simulink model "Sat_Int_test"  (Simulink 7.3)
settings: Solver=ode45  StartTime=0.0  StopTime=10.0  RelTol=1e-3
settings Model: Creator=MD710  LastModifiedBy=MD710
settings DebuggingCC: SaveWithParameterizedLinksMsg=none  SolverPrmCheckMsg=none  MultiTaskDSMMsg=warning  MultiTaskCondExecSysMsg=none  FcnCallInpInsideContextMsg=Enable All  StrictBusMsg=None
settings HardwareCC: TargetHWDeviceType=32-bit Generic
settings RTWCC: IncludeERTFirstTime=on
settings GRTTargetCC: TargetFcnLib=ansi_tfl_tmw.mat

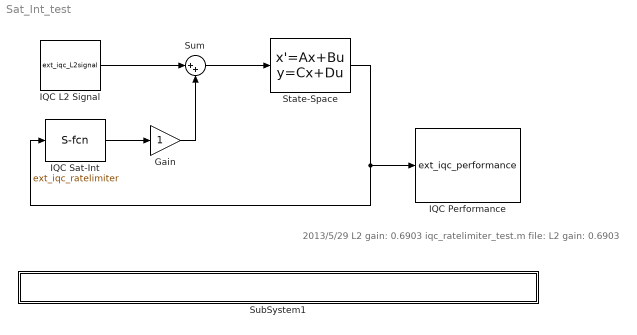
== system Sat_Int_test ==
  note: 2013/5/29 L2 gain: 0.6903
      | iqc_ratelimiter_test.m file: L2 gain: 0.6903
  Gain : Gain
  IQC L2 Signal : M-S-Function  FunctionName=ext_iqc_L2signal  Parameters=sig_size,sam_time,sig_type,tru_time,sig_amp,sig_fre,user_cus  mask(IQC L2 signal(ver:0.1)){sig_size=1, sam_time=0, sig_type=Step, tru_time=10, sig_amp=1, sig_fre=1, user_cus='2*exp(3*t)'}
      mask prompts: sig_size "Signal Dimension:(Default: 1)"; sam_time "Sample Time:(Default: 0)"; sig_type "Signal Type:"; tru_time "Truncation Time:"; sig_amp "Maximum Amplitude:"; sig_fre "Frequency:"; user_cus "Custom:"
      mask help:
      | Important:
      | In IQC procedure step (as commond iqc_gain_tbx, the task is get
      | L2 gain value), regardless of the user to choose which option (ex sine...),
      | here regarded as generalized L2 signal.
      mask StyleString: edit,edit,popup(Step|Square wave|Sine wave|Custom|Random|External),edit,edit,edit,edit
      mask CallbackString: ||iqc_block_cho(gcb,'L2signal_type')||||
      mask TabNameString: Generalized Parameters,Generalized Parameters,Simulink Parameters,Simulink Parameters,Simulink Parameters,Simulink Parameters,Simulink Parameters
      mask Display: plot(0:0.1:10,[sin(0:0.1:6.2) zeros(1,38)])
  IQC Performance : M-S-Function  FunctionName=ext_iqc_performance  Parameters=imp_met,save_lin_com,isiqcbode,fre_ran,uselmitool,lmi_par  mask(IQC Performance(ver:0.1)){imp_met=Only Calculation, save_lin_com=off, isiqcbode=off, fre_ran='', uselmitool=lmilab, lmi_par=''}
      mask prompts: imp_met "Implementation Methods"; save_lin_com "Save the Linear File and Command File"; isiqcbode "Display IQC Bode Figure"; fre_ran "Frequency Range:(Default: empty)"; uselmitool "LMI Tool:"; lmi_par "Parameter:(if empty use define)"
      mask help:
      | Important:
      | In IQC toolbox calculate step (as commond iqc_gain_tbx, the task is get
      | L2 gain value), regardless of the user to connect any signal input(Even if
      | not a signal), here regarded as generalized L2 signal.
      |
      | Example 1: setlmioptions('',[0 200 0 0 777])
      | the block parameter is
      | LMI Tool: lmilab
      | Parameter:
      |        [0 200 0 0 777]
      |
      | Example 2: setlmioptions('yalmip','solver','sdpt3','verbose',1)
      | the block parameter is
      | LMI Tool: yalmip
      | Parameter:
      |        {'solver',sdpt3','verbose',1}
      mask Help:
      | <a href="matlab:doc abst_init_iqc;">abst_init_iqc</a>
      | <a href="matlab:doc setlmioptions;">setlmioptions</a>
      | <a href="matlab:doc iqc_gain_tbx;">iqc_gain_tbx</a>
      mask StyleString: popup(Calculation and Simulation|Only Calculation|Only Simulation),checkbox,checkbox,edit,popup(lmilab|yalmip),edit
      mask CallbackString: iqc_block_cho(gcb,'performance_imp')||iqc_block_cho(gcb,'performance_bodefre')|||
      mask TabNameString: Parameter,Parameter,Parameter,Parameter,LMI Parameter,LMI Parameter
      mask Display: fprintf('In -> Out \n performance \n L2 gain:\n%4.4f',0.69027);
  IQC Sat-Int : M-S-Function  FunctionName=ext_iqc_ratelimiter  Parameters=pole,k,out_var  mask(IQC Sat-Int(ver:0.1)){pole=[1,1], k=1, out_var=''}
      mask prompts: pole "Pole:(Default: [1,1])"; k "d(sat(0))/dt Value:(Default: 1)"; out_var "Output Variable:(Default: empty)"
      mask help:
      | Example: [w,M]=iqc_ratelimiter(v,a,k)
      | Pole:
      |     [a]
      | d(sat(0))/dt Value:
      |      k
      | Output Variable:
      |     {'M'}
      mask Help: eval('doc iqc_ratelimiter')
      mask Display: plot(0,0,100,100,[18,45,45,18,18],[60,60,26,26,60],[62,82,82,62,62],[60,60,26,26,60],[62,0],[44,44],[79,65],[44,44],[71,71],[46,57],[68,69,72,74,73,71,69,68,69,72,74],[31,29,29,31,34,35,36,38,40,40,39],[31,31],[26,60],[45,38,24],[55,55,33],[24,18],[33,33],[99,82],[44,44],[10,12,8,10,10,90,90],[44,51,51,44,80,80,44],[7,2],[55,55]);
  State-Space : StateSpace  A=[-5,1;2,-3]  B=[0;1]  C=[0 1]  D=[0]
  SubSystem1 : Subsystem  mask{filename=iqc_ratelimiter_test.m}
      mask init:
      | x_dir=which(filename);
      | x=x_dir;
      settings: OpenFcn=|
      | x_dir=which('iqc_ratelimiter_test.m');
      | x=x_dir;
      | edit(x);
      mask Display: disp(['MATLAB file: ' x]);
  Sum : Sum  Inputs=|++
  wires:
  Sum/1 -> State-Space/1
  IQC Sat-Int/1 -> Gain/1
  Gain/1 -> Sum/2
  IQC L2 Signal/1 -> Sum/1
  State-Space/1 -> IQC Performance/1, IQC Sat-Int/1

== system Sat_Int_test/SubSystem1 ==
